simulink model "veh_passenger_simulation"  (R2018b)
settings: Solver=ode2  StartTime=0.0  StopTime=200  FixedStep=0.002  RelTol=1e-3  EnableMultiTasking=on
model workspace (MAT data in the model file):
  m = 1000
undefined symbols (not defined in the file or in its folder): tSPhysics, TUMHealthStatus, TUMVehicleState, veh_param, veh_param_db, x0_positionstates, x0_vehiclepose
libraries: general_sensor_lib x12, simulink x1, rr_general x1
settings Model: DataDictionary=veh_passenger_simulation.sldd  PauseTimes=9.280  Creator=wischnewski  LastModifiedBy=ge34qer
settings DataIOCC: SaveFormat=StructureWithTime
settings OptimizationCC: BlockReduction=off  DefaultParameterBehavior=Inlined  OptimizeBlockIOStorage=off  BufferReuse=off  GlobalBufferReuse=off  ExpressionFolding=off  LocalBlockOutputs=off  LifeSpan=inf  OptimizeDataStoreBuffers=off  BusAssignmentInplaceUpdate=off
settings HardwareCC: ProdBitPerPointer=32  ProdBitPerSizeT=32  ProdBitPerPtrDiffT=32  ProdLargestAtomicFloat=None  ProdWordSize=32  ProdLongLongMode=on  ProdHWDeviceType=Generic->32-bit x86 compatible
settings ModelReferenceCC: ModelReferenceMinAlgLoopOccurrences=on
settings SFSimCC: SimUseLocalCustomCode=off
settings RTWCC: Description=Generic Real-Time Target  GenerateReport=on  RTWUseLocalCustomCode=off  LaunchReport=on
settings CodeAppCC: ForceParamTrailComments=on  OperatorAnnotations=on  StateflowObjectComments=on  MATLABSourceComments=on
settings GRTTargetCC: TargetLangStandard=C89/C90 (ANSI)

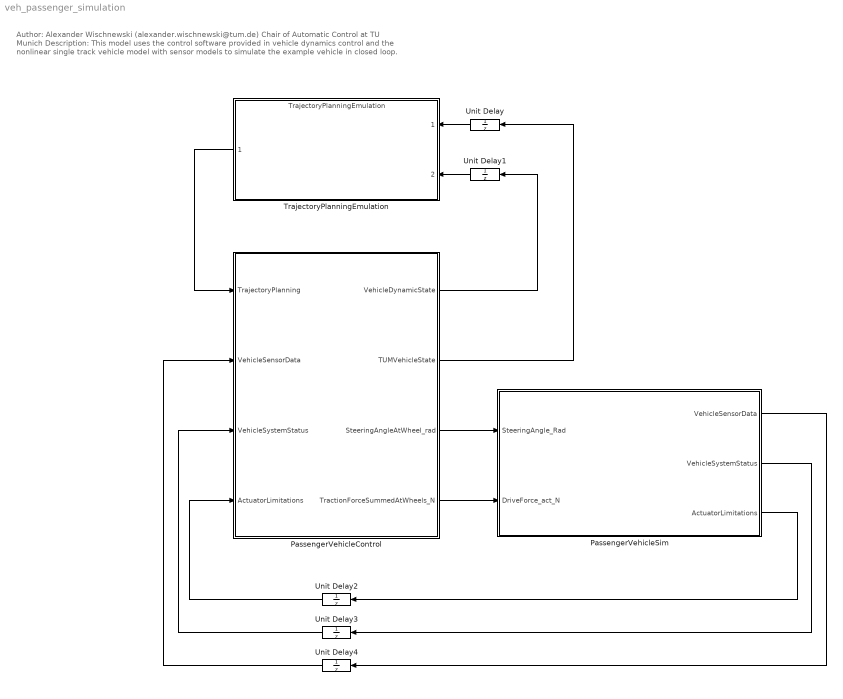
== system veh_passenger_simulation ==
  note: Author: Alexander Wischnewski (alexander.wischnewski@tum.de)
      | Chair of Automatic Control at TU Munich
      |
      | Description: This model uses the control software provided in vehicle dynamics control and the nonlinear single track vehicle model
      | with sensor models to simulate the example vehicle in closed loop.
  PassengerVehicleControl : Subsystem
  PassengerVehicleSim : Subsystem
  TrajectoryPlanningEmulation : ModelReference  ModelNameDialog=TrajectoryPlanningEmulation.slx  ParameterArgumentNames=Raceline  ParameterArgumentValues=Raceline  UsingDefaultArgumentValue=0  SimulationMode=Normal  ModelReferenceVersion=1.667
  Unit Delay : UnitDelay  InitialCondition=TUMVehicleState.OFF  SampleTime=-1
  Unit Delay{1..4} (4 alike) : UnitDelay  SampleTime=-1
  wires:
  PassengerVehicleControl/3(SteeringAngleAtWheel_rad) -> PassengerVehicleSim/1(SteeringAngle_Rad)
  PassengerVehicleControl/4(TractionForceSummedAtWheels_N) -> PassengerVehicleSim/2(DriveForce_act_N)
  TrajectoryPlanningEmulation/1 -> PassengerVehicleControl/1(TrajectoryPlanning)
  PassengerVehicleControl/1(VehicleDynamicState) -> Unit Delay1/1
  PassengerVehicleControl/2(TUMVehicleState) -> Unit Delay/1
  Unit Delay/1 -> TrajectoryPlanningEmulation/1
  Unit Delay1/1 -> TrajectoryPlanningEmulation/2
  PassengerVehicleSim/3(ActuatorLimitations) -> Unit Delay2/1
  Unit Delay2/1 -> PassengerVehicleControl/4(ActuatorLimitations)
  PassengerVehicleSim/2(VehicleSystemStatus) -> Unit Delay3/1
  Unit Delay3/1 -> PassengerVehicleControl/3(VehicleSystemStatus)
  PassengerVehicleSim/1(VehicleSensorData) -> Unit Delay4/1
  Unit Delay4/1 -> PassengerVehicleControl/2(VehicleSensorData)

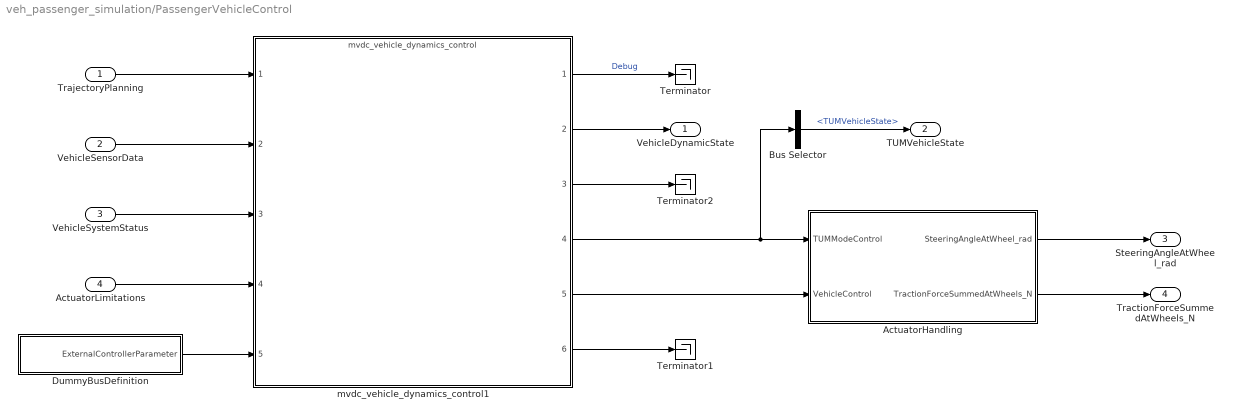
== system veh_passenger_simulation/PassengerVehicleControl ==
  TrajectoryPlanning : Inport
  VehicleSensorData : Inport  Port=2
  VehicleSystemStatus : Inport  Port=3
  ActuatorLimitations : Inport  Port=4
  ActuatorHandling : Subsystem
  Bus Selector : BusSelector  OutputSignals=TUMVehicleState
  DummyBusDefinition : Subsystem
  Terminator : Terminator
  Terminator1 : Terminator
  Terminator2 : Terminator
  mvdc_vehicle_dynamics_control1 : ModelReference  ModelNameDialog=mvdc_vehicle_dynamics_control  SimulationMode=Normal  ModelReferenceVersion=1.726
  VehicleDynamicState : Outport
  TUMVehicleState : Outport  Port=2
  SteeringAngleAtWheel_rad : Outport  Port=3
  TractionForceSummedAtWheels_N : Outport  Port=4
  wires:
  mvdc_vehicle_dynamics_control1/1 -> Terminator/1  "Debug"
  VehicleSystemStatus/1 -> mvdc_vehicle_dynamics_control1/3
  ActuatorLimitations/1 -> mvdc_vehicle_dynamics_control1/4
  VehicleSensorData/1 -> mvdc_vehicle_dynamics_control1/2
  TrajectoryPlanning/1 -> mvdc_vehicle_dynamics_control1/1
  mvdc_vehicle_dynamics_control1/5 -> ActuatorHandling/2(VehicleControl)
  mvdc_vehicle_dynamics_control1/4 -> Bus Selector/1, ActuatorHandling/1(TUMModeControl)
  mvdc_vehicle_dynamics_control1/6 -> Terminator1/1
  mvdc_vehicle_dynamics_control1/3 -> Terminator2/1
  mvdc_vehicle_dynamics_control1/2 -> VehicleDynamicState/1
  ActuatorHandling/2(TractionForceSummedAtWheels_N) -> TractionForceSummedAtWheels_N/1
  ActuatorHandling/1(SteeringAngleAtWheel_rad) -> SteeringAngleAtWheel_rad/1
  DummyBusDefinition/1(ExternalControllerParameter) -> mvdc_vehicle_dynamics_control1/5
  Bus Selector/1 -> TUMVehicleState/1  "<TUMVehicleState>"

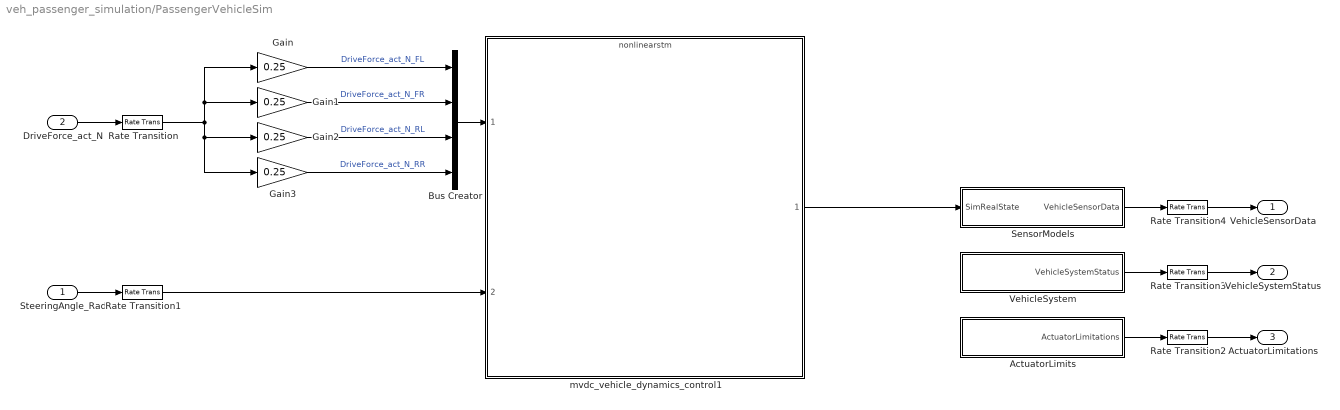
== system veh_passenger_simulation/PassengerVehicleSim ==
  SteeringAngle_Rad : Inport
  DriveForce_act_N : Inport  Port=2
  ActuatorLimits : Subsystem
  Bus Creator : BusCreator  Inputs=4
  Gain{,1..3} (4 alike) : Gain  Gain=0.25
  Rate Transition{,1..4} (5 alike) : RateTransition
  SensorModels : Subsystem
  VehicleSystem : Subsystem
  mvdc_vehicle_dynamics_control1 : ModelReference  ModelNameDialog=nonlinearstm.slx  ParameterArgumentNames=veh_param,x0_positionstates  ParameterArgumentValues=veh_param_db,x0_vehiclepose  UsingDefaultArgumentValue=0,0  SimulationMode=Normal  ModelReferenceVersion=1.284
  VehicleSensorData : Outport
  VehicleSystemStatus : Outport  Port=2
  ActuatorLimitations : Outport  Port=3
  wires:
  SteeringAngle_Rad/1 -> Rate Transition1/1
  Bus Creator/1 -> mvdc_vehicle_dynamics_control1/1
  Gain3/1 -> Bus Creator/4  "DriveForce_act_N_RR"
  Gain2/1 -> Bus Creator/3  "DriveForce_act_N_RL"
  Gain1/1 -> Bus Creator/2  "DriveForce_act_N_FR"
  Gain/1 -> Bus Creator/1  "DriveForce_act_N_FL"
  DriveForce_act_N/1 -> Rate Transition/1
  ActuatorLimits/1(ActuatorLimitations) -> Rate Transition2/1
  VehicleSystem/1(VehicleSystemStatus) -> Rate Transition3/1
  mvdc_vehicle_dynamics_control1/1 -> SensorModels/1(SimRealState)
  SensorModels/1(VehicleSensorData) -> Rate Transition4/1
  Rate Transition/1 -> Gain1/1, Gain/1, Gain3/1, Gain2/1
  Rate Transition1/1 -> mvdc_vehicle_dynamics_control1/2
  Rate Transition2/1 -> ActuatorLimitations/1
  Rate Transition3/1 -> VehicleSystemStatus/1
  Rate Transition4/1 -> VehicleSensorData/1

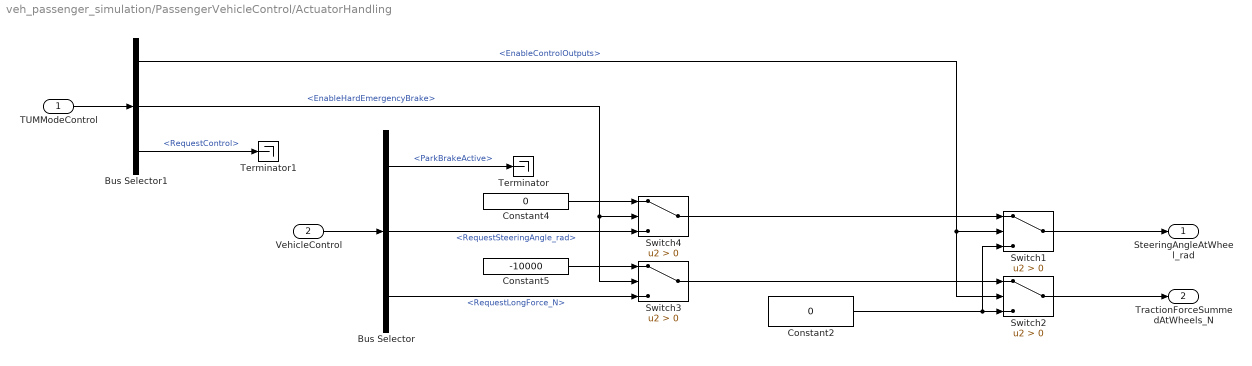
== system veh_passenger_simulation/PassengerVehicleControl/ActuatorHandling ==
  TUMModeControl : Inport  OutDataTypeStr=Bus: TUMModeControl
  VehicleControl : Inport  Port=2  OutDataTypeStr=Bus: VehicleControl
  Bus Selector : BusSelector  OutputSignals=ParkBrakeActive,RequestSteeringAngle_rad,RequestLongForce_N
  Bus Selector1 : BusSelector  OutputSignals=EnableControlOutputs,EnableHardEmergencyBrake,RequestControl
  Constant2 : Constant  Value=0
  Constant4 : Constant  Value=0
  Constant5 : Constant  Value=-10000
  Switch{1..4} (4 alike) : Switch  Criteria=u2 > Threshold
  Terminator : Terminator
  Terminator1 : Terminator
  SteeringAngleAtWheel_rad : Outport
  TractionForceSummedAtWheels_N : Outport  Port=2
  wires:
  Bus Selector1/1 -> Switch2/2, Switch1/2  "<EnableControlOutputs>"
  TUMModeControl/1 -> Bus Selector1/1
  Bus Selector/3 -> Switch3/3  "<RequestLongForce_N>"
  Constant2/1 -> Switch1/3, Switch2/3
  VehicleControl/1 -> Bus Selector/1
  Bus Selector/2 -> Switch4/3  "<RequestSteeringAngle_rad>"
  Constant4/1 -> Switch4/1
  Constant5/1 -> Switch3/1
  Bus Selector1/2 -> Switch3/2, Switch4/2  "<EnableHardEmergencyBrake>"
  Bus Selector/1 -> Terminator/1  "<ParkBrakeActive>"
  Bus Selector1/3 -> Terminator1/1  "<RequestControl>"
  Switch4/1 -> Switch1/1
  Switch3/1 -> Switch2/1
  Switch1/1 -> SteeringAngleAtWheel_rad/1
  Switch2/1 -> TractionForceSummedAtWheels_N/1

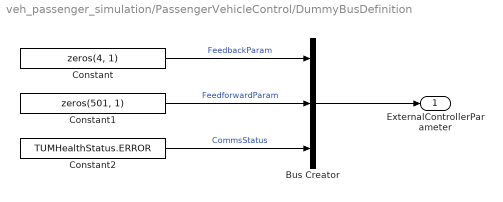
== system veh_passenger_simulation/PassengerVehicleControl/DummyBusDefinition ==
  Bus Creator : BusCreator  Inputs=3
  Constant : Constant  Value=zeros(4, 1)
  Constant1 : Constant  Value=zeros(501, 1)
  Constant2 : Constant  Value=TUMHealthStatus.ERROR
  ExternalControllerParameter : Outport
  wires:
  Bus Creator/1 -> ExternalControllerParameter/1
  Constant/1 -> Bus Creator/1  "FeedbackParam"
  Constant1/1 -> Bus Creator/2  "FeedforwardParam"
  Constant2/1 -> Bus Creator/3  "CommsStatus"

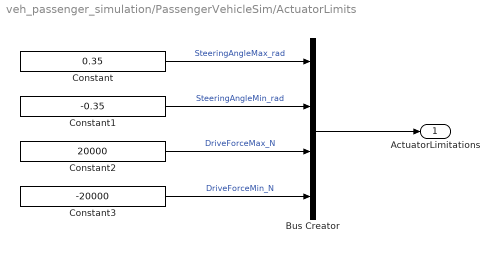
== system veh_passenger_simulation/PassengerVehicleSim/ActuatorLimits ==
  Bus Creator : BusCreator  Inputs=4
  Constant : Constant  Value=0.35
  Constant1 : Constant  Value=-0.35
  Constant2 : Constant  Value=20000
  Constant3 : Constant  Value=-20000
  ActuatorLimitations : Outport
  wires:
  Bus Creator/1 -> ActuatorLimitations/1
  Constant/1 -> Bus Creator/1  "SteeringAngleMax_rad"
  Constant1/1 -> Bus Creator/2  "SteeringAngleMin_rad"
  Constant2/1 -> Bus Creator/3  "DriveForceMax_N"
  Constant3/1 -> Bus Creator/4  "DriveForceMin_N"

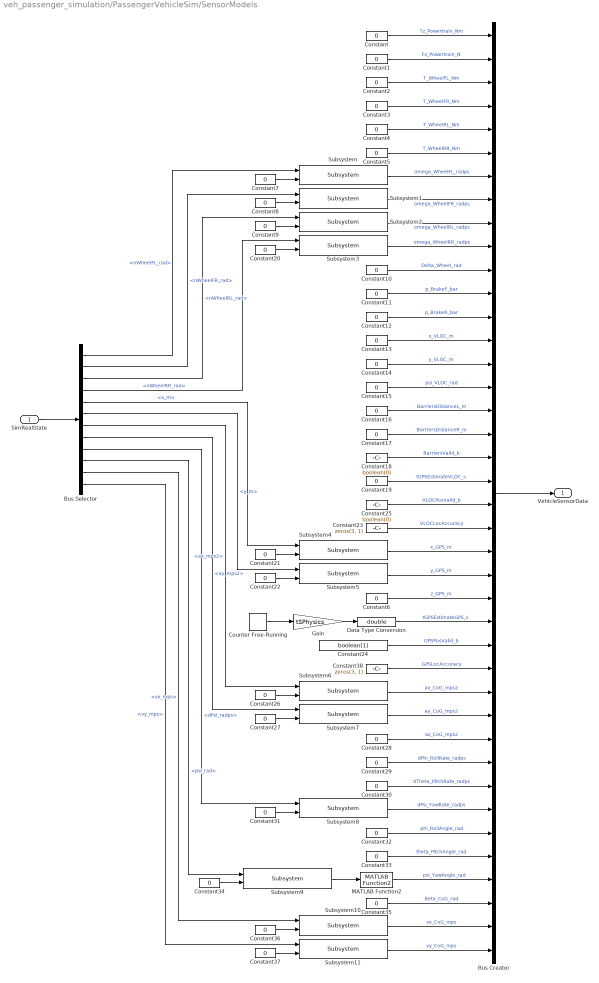
== system veh_passenger_simulation/PassengerVehicleSim/SensorModels ==
  SimRealState : Inport
  Bus Creator : BusCreator  Inputs=40
  Bus Selector : BusSelector  OutputSignals=nWheelFL_rad,nWheelFR_rad,nWheelRL_rad,nWheelRR_rad,x_m,y_m,ax_mps2,ay_mps2,dPsi_radps,psi_rad,vx_mps,vy_mps
  Constant{,1..17,19..22,26..37} (34 alike) : Constant  Value=0
  Constant18 : Constant  Value=boolean(0)
  Constant23 : Constant  Value=zeros(3, 1)
  Constant24 : Constant  Value=boolean(1)
  Constant25 : Constant  Value=boolean(0)
  Constant38 : Constant  Value=zeros(3, 1)
  Counter Free-Running : simulink/Sources/Counter Free-Running  NumBits=32  tsamp=tSPhysics
  Data Type Conversion : DataTypeConversion  OutDataTypeStr=double
  Gain : Gain  Gain=tSPhysics
  MATLAB Function2 : rr_general/MATLAB Function2  SystemSampleTime=-1
  Subsystem{,1..3,6..7} (6 alike) : general_sensor_lib/Subsystem  Noise=0.1  Delay=0  SampleRate=tSPhysics
  Subsystem10 : general_sensor_lib/Subsystem  Noise=0.01  Delay=0  SampleRate=tSPhysics
  Subsystem11 : general_sensor_lib/Subsystem  Noise=0.01  Delay=0  SampleRate=tSPhysics
  Subsystem{4..5,8..9} (4 alike) : general_sensor_lib/Subsystem  Noise=0.001  Delay=0  SampleRate=tSPhysics
  VehicleSensorData : Outport
  wires:
  Bus Creator/1 -> VehicleSensorData/1
  Constant/1 -> Bus Creator/1  "Tz_Powertrain_Nm"
  Constant1/1 -> Bus Creator/2  "Fx_Powertrain_N"
  Constant2/1 -> Bus Creator/3  "T_WheelFL_Nm"
  Constant3/1 -> Bus Creator/4  "T_WheelFR_Nm"
  Constant4/1 -> Bus Creator/5  "T_WheelRL_Nm"
  Constant5/1 -> Bus Creator/6  "T_WheelRR_Nm"
  Subsystem/1 -> Bus Creator/7  "omega_WheelFL_radps"
  Subsystem1/1 -> Bus Creator/8  "omega_WheelFR_radps"
  Subsystem2/1 -> Bus Creator/9  "omega_WheelRL_radps"
  Subsystem3/1 -> Bus Creator/10  "omega_WheelRR_radps"
  Constant10/1 -> Bus Creator/11  "Delta_Wheel_rad"
  Constant11/1 -> Bus Creator/12  "p_BrakeF_bar"
  Constant12/1 -> Bus Creator/13  "p_BrakeR_bar"
  Constant13/1 -> Bus Creator/14  "x_VLOC_m"
  Constant14/1 -> Bus Creator/15  "y_VLOC_m"
  Constant15/1 -> Bus Creator/16  "psi_VLOC_rad"
  Constant16/1 -> Bus Creator/17  "BarriersDistanceL_m"
  Constant17/1 -> Bus Creator/18  "BarriersDistanceR_m"
  Constant18/1 -> Bus Creator/19  "BarriersValid_b"
  Constant19/1 -> Bus Creator/20  "tGPSEstimateVLOC_s"
  Subsystem4/1 -> Bus Creator/23  "x_GPS_m"
  Subsystem5/1 -> Bus Creator/24  "y_GPS_m"
  Constant6/1 -> Bus Creator/25  "z_GPS_m"
  Gain/1 -> Data Type Conversion/1
  Constant24/1 -> Bus Creator/27  "GPSPosValid_b"
  Constant25/1 -> Bus Creator/21  "VLOCPosValid_b"
  Subsystem6/1 -> Bus Creator/29  "ax_CoG_mps2"
  Subsystem7/1 -> Bus Creator/30  "ay_CoG_mps2"
  Constant28/1 -> Bus Creator/31  "az_CoG_mps2"
  Constant29/1 -> Bus Creator/32  "dPhi_RollRate_radps"
  Constant30/1 -> Bus Creator/33  "dTheta_PitchRate_radps"
  Subsystem8/1 -> Bus Creator/34  "dPsi_YawRate_radps"
  Constant32/1 -> Bus Creator/35  "phi_RollAngle_rad"
  Constant33/1 -> Bus Creator/36  "theta_PitchAngle_rad"
  Subsystem9/1 -> MATLAB Function2/1
  Constant35/1 -> Bus Creator/38  "Beta_CoG_rad"
  Subsystem10/1 -> Bus Creator/39  "vx_CoG_mps"
  Subsystem11/1 -> Bus Creator/40  "vy_CoG_mps"
  SimRealState/1 -> Bus Selector/1
  Bus Selector/1 -> Subsystem/1  "<nWheelFL_rad>"
  Bus Selector/2 -> Subsystem1/1  "<nWheelFR_rad>"
  Bus Selector/3 -> Subsystem2/1  "<nWheelRL_rad>"
  Bus Selector/4 -> Subsystem3/1  "<nWheelRR_rad>"
  Bus Selector/5 -> Subsystem4/1  "<x_m>"
  Bus Selector/6 -> Subsystem5/1  "<y_m>"
  Bus Selector/7 -> Subsystem6/1  "<ax_mps2>"
  Bus Selector/8 -> Subsystem7/1  "<ay_mps2>"
  Bus Selector/9 -> Subsystem8/1  "<dPsi_radps>"
  Bus Selector/11 -> Subsystem10/1  "<vx_mps>"
  Bus Selector/12 -> Subsystem11/1  "<vy_mps>"
  Constant7/1 -> Subsystem/2
  Constant8/1 -> Subsystem1/2
  Constant9/1 -> Subsystem2/2
  Constant20/1 -> Subsystem3/2
  Constant21/1 -> Subsystem4/2
  Constant22/1 -> Subsystem5/2
  Constant26/1 -> Subsystem6/2
  Constant27/1 -> Subsystem7/2
  Constant31/1 -> Subsystem8/2
  Constant34/1 -> Subsystem9/2
  Constant36/1 -> Subsystem10/2
  Constant37/1 -> Subsystem11/2
  Counter Free-Running/1 -> Gain/1
  Data Type Conversion/1 -> Bus Creator/26  "tGPSEstimateGPS_s"
  Bus Selector/10 -> Subsystem9/1  "<psi_rad>"
  MATLAB Function2/1 -> Bus Creator/37  "psi_YawAngle_rad"
  Constant23/1 -> Bus Creator/22  "VLOCLocAccuracy"
  Constant38/1 -> Bus Creator/28  "GPSLocAccuracy"

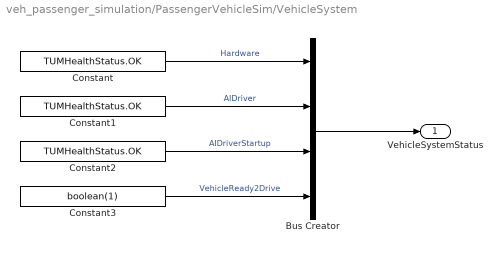
== system veh_passenger_simulation/PassengerVehicleSim/VehicleSystem ==
  Bus Creator : BusCreator  Inputs=4
  Constant : Constant  Value=TUMHealthStatus.OK
  Constant1 : Constant  Value=TUMHealthStatus.OK
  Constant2 : Constant  Value=TUMHealthStatus.OK
  Constant3 : Constant  Value=boolean(1)
  VehicleSystemStatus : Outport
  wires:
  Bus Creator/1 -> VehicleSystemStatus/1
  Constant/1 -> Bus Creator/1  "Hardware"
  Constant1/1 -> Bus Creator/2  "AIDriver"
  Constant2/1 -> Bus Creator/3  "AIDriverStartup"
  Constant3/1 -> Bus Creator/4  "VehicleReady2Drive"
